simulink model "EHB_MOTOR"  (R2023b)
settings: Solver=FixedStepDiscrete  StartTime=0.0  StopTime=inf  FixedStep=0.0001  RelTol=1e-3  EnableMultiTasking=on
undefined symbols (not defined in the file): CAN_EHB_VCU0x125, CAN_EHB_VCU0x126, CAN_id0x120_Data, Cos_Table, Cos_Table1, EHB_DTC_status, R, Sin_BreakPoint, Sin_BreakPoint1, Sin_Table, Sin_Table1, T
libraries: simulink x30
(part 3 of 9)

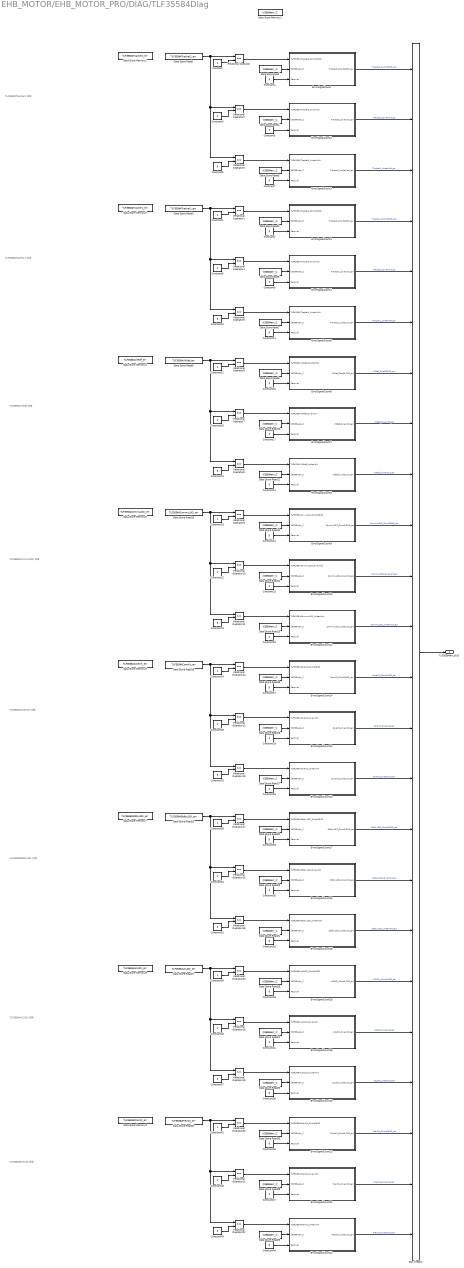
== system EHB_MOTOR/EHB_MOTOR_PRO/DIAG/TLF35584Diag ==
  note: TLF35584Tracker2故障
  note: TLF35584Tracker1故障
  note: TLF35584VltRef故障
  note: TLF35584CommuLDO故障
  note: TLF35584CoreVolt故障
  note: TLF35584StdbyLDO故障
  note: TLF35584uCLDO故障
  note: TLF35584PreVolt故障
  Bus Creator : BusCreator  Inputs=24
  Constant{,1,12,18,24,30,36,42} (8 alike) : Constant
  Constant{6,10,13,19,25,31,37,43} (8 alike) : Constant  Value=3
  Constant{2,4..5,7,9,11,14..15,17,20..21,23,26..27,29,32..33,35,38..39,41,44..45,47} (24 alike) : Constant  Value=0  OutDataTypeStr=uint8
  Constant{3,8,16,22,28,34,40,46} (8 alike) : Constant  Value=2
  Data Store Memory1 : DataStoreMemory  DataStoreName=ti35584err_C  ReadBeforeWriteMsg=warning  WriteAfterWriteMsg=warning  WriteAfterReadMsg=warning  ShowAdditionalParam=off  OutDataTypeStr=uint16
  Data Store Memory2 : DataStoreMemory  DataStoreName=TLF35584Tracker2_err  ReadBeforeWriteMsg=warning  WriteAfterWriteMsg=warning  WriteAfterReadMsg=warning  ShowAdditionalParam=off  OutDataTypeStr=uint8
  Data Store Memory3 : DataStoreMemory  DataStoreName=TLF35584Tracker1_err  ReadBeforeWriteMsg=warning  WriteAfterWriteMsg=warning  WriteAfterReadMsg=warning  ShowAdditionalParam=off  OutDataTypeStr=uint8
  Data Store Memory4 : DataStoreMemory  DataStoreName=TLF35584VltRef_err  ReadBeforeWriteMsg=warning  WriteAfterWriteMsg=warning  WriteAfterReadMsg=warning  ShowAdditionalParam=off  OutDataTypeStr=uint8
  Data Store Memory5 : DataStoreMemory  DataStoreName=TLF35584CommuLDO_err  ReadBeforeWriteMsg=warning  WriteAfterWriteMsg=warning  WriteAfterReadMsg=warning  ShowAdditionalParam=off  OutDataTypeStr=uint8
  Data Store Memory6 : DataStoreMemory  DataStoreName=TLF35584CoreVlt_err  ReadBeforeWriteMsg=warning  WriteAfterWriteMsg=warning  WriteAfterReadMsg=warning  ShowAdditionalParam=off  OutDataTypeStr=uint8
  Data Store Memory7 : DataStoreMemory  DataStoreName=TLF35584StdbyLDO_err  ReadBeforeWriteMsg=warning  WriteAfterWriteMsg=warning  WriteAfterReadMsg=warning  ShowAdditionalParam=off  OutDataTypeStr=uint8
  Data Store Memory8 : DataStoreMemory  DataStoreName=TLF35584uCLDO_err  ReadBeforeWriteMsg=warning  WriteAfterWriteMsg=warning  WriteAfterReadMsg=warning  ShowAdditionalParam=off  OutDataTypeStr=uint8
  Data Store Memory9 : DataStoreMemory  DataStoreName=TLF35584PreVolt_err  ReadBeforeWriteMsg=warning  WriteAfterWriteMsg=warning  WriteAfterReadMsg=warning  ShowAdditionalParam=off  OutDataTypeStr=uint8
  Data Store Read{,2,4..8,10..14,16..18,20..22,24..26,28..30} (24 alike) : DataStoreRead  DataStoreName=ti35584err_C  DataStoreElements=ti35584err_C  IndexOptions=Index vector (dialog)  Indices=1  OutputSizes=1
  Data Store Read1 : DataStoreRead  DataStoreName=TLF35584Tracker2_err  DataStoreElements=TLF35584Tracker2_err  IndexOptions=Index vector (dialog)  Indices=1  OutputSizes=1
  Data Store Read15 : DataStoreRead  DataStoreName=TLF35584CommuLDO_err  DataStoreElements=TLF35584CommuLDO_err  IndexOptions=Index vector (dialog)  Indices=1  OutputSizes=1
  Data Store Read19 : DataStoreRead  DataStoreName=TLF35584CoreVlt_err  DataStoreElements=TLF35584CoreVlt_err  IndexOptions=Index vector (dialog)  Indices=1  OutputSizes=1
  Data Store Read23 : DataStoreRead  DataStoreName=TLF35584StdbyLDO_err  DataStoreElements=TLF35584StdbyLDO_err  IndexOptions=Index vector (dialog)  Indices=1  OutputSizes=1
  Data Store Read27 : DataStoreRead  DataStoreName=TLF35584uCLDO_err  DataStoreElements=TLF35584uCLDO_err  IndexOptions=Index vector (dialog)  Indices=1  OutputSizes=1
  Data Store Read3 : DataStoreRead  DataStoreName=TLF35584Tracker1_err  DataStoreElements=TLF35584Tracker1_err  IndexOptions=Index vector (dialog)  Indices=1  OutputSizes=1
  Data Store Read31 : DataStoreRead  DataStoreName=TLF35584PreVolt_err  DataStoreElements=TLF35584PreVolt_err  IndexOptions=Index vector (dialog)  Indices=1  OutputSizes=1
  Data Store Read9 : DataStoreRead  DataStoreName=TLF35584VltRef_err  DataStoreElements=TLF35584VltRef_err  IndexOptions=Index vector (dialog)  Indices=1  OutputSizes=1
  ErrorSignalCount : Stateflow chart  TreatAsAtomicUnit=on
  ErrorSignalCount1 : Stateflow chart  TreatAsAtomicUnit=on
  ErrorSignalCount10 : Stateflow chart  TreatAsAtomicUnit=on
  ErrorSignalCount11 : Stateflow chart  TreatAsAtomicUnit=on
  ErrorSignalCount12 : Stateflow chart  TreatAsAtomicUnit=on
  ErrorSignalCount13 : Stateflow chart  TreatAsAtomicUnit=on
  ErrorSignalCount14 : Stateflow chart  TreatAsAtomicUnit=on
  ErrorSignalCount15 : Stateflow chart  TreatAsAtomicUnit=on
  ErrorSignalCount16 : Stateflow chart  TreatAsAtomicUnit=on
  ErrorSignalCount17 : Stateflow chart  TreatAsAtomicUnit=on
  ErrorSignalCount18 : Stateflow chart  TreatAsAtomicUnit=on
  ErrorSignalCount19 : Stateflow chart  TreatAsAtomicUnit=on
  ErrorSignalCount2 : Stateflow chart  TreatAsAtomicUnit=on
  ErrorSignalCount20 : Stateflow chart  TreatAsAtomicUnit=on
  ErrorSignalCount21 : Stateflow chart  TreatAsAtomicUnit=on
  ErrorSignalCount22 : Stateflow chart  TreatAsAtomicUnit=on
  ErrorSignalCount23 : Stateflow chart  TreatAsAtomicUnit=on
  ErrorSignalCount3 : Stateflow chart  TreatAsAtomicUnit=on
  ErrorSignalCount4 : Stateflow chart  TreatAsAtomicUnit=on
  ErrorSignalCount5 : Stateflow chart  TreatAsAtomicUnit=on
  ErrorSignalCount6 : Stateflow chart  TreatAsAtomicUnit=on
  ErrorSignalCount7 : Stateflow chart  TreatAsAtomicUnit=on
  ErrorSignalCount8 : Stateflow chart  TreatAsAtomicUnit=on
  ErrorSignalCount9 : Stateflow chart  TreatAsAtomicUnit=on
  Relational Operator{,1..23} (24 alike) : RelationalOperator  Operator===  OutDataTypeStr=boolean  RndMeth=Simplest  InputSameDT=off
  TLF35584err_BUS : Outport  VectorParamsAs1DForOutWhenUnconnected=off
  wires:
  Data Store Read/1 -> ErrorSignalCount/2(ti35584err_C)
  Constant4/1 -> ErrorSignalCount/3(Recover)
  Data Store Read1/1 -> Relational Operator/1, Relational Operator2/1, Relational Operator3/1
  Constant/1 -> Relational Operator/2
  Relational Operator/1 -> ErrorSignalCount/1(TLF35584Tracker2_Short2GND)
  Relational Operator1/1 -> ErrorSignalCount1/1(TLF35584Tracker1_Short2GND)
  Constant1/1 -> Relational Operator1/2
  Constant2/1 -> ErrorSignalCount1/3(Recover)
  Data Store Read2/1 -> ErrorSignalCount1/2(ti35584err_C)
  Constant3/1 -> Relational Operator2/2
  Constant5/1 -> ErrorSignalCount2/3(Recover)
  Data Store Read4/1 -> ErrorSignalCount2/2(ti35584err_C)
  Relational Operator2/1 -> ErrorSignalCount2/1(TLF35584Tracker2_OverVolt)
  Constant6/1 -> Relational Operator3/2
  Relational Operator3/1 -> ErrorSignalCount3/1(TLF35584Tracker2_UnderVolt)
  Data Store Read5/1 -> ErrorSignalCount3/2(ti35584err_C)
  Constant7/1 -> ErrorSignalCount3/3(Recover)
  Constant11/1 -> ErrorSignalCount5/3(Recover)
  Data Store Read7/1 -> ErrorSignalCount5/2(ti35584err_C)
  Relational Operator5/1 -> ErrorSignalCount5/1(TLF35584Tracker1_UnderVolt)
  Constant10/1 -> Relational Operator5/2
  Relational Operator4/1 -> ErrorSignalCount4/1(TLF35584Tracker1_OverVolt)
  Data Store Read6/1 -> ErrorSignalCount4/2(ti35584err_C)
  Constant9/1 -> ErrorSignalCount4/3(Recover)
  Constant8/1 -> Relational Operator4/2
  Data Store Read3/1 -> Relational Operator5/1, Relational Operator4/1, Relational Operator1/1
  Data Store Read9/1 -> Relational Operator6/1, Relational Operator7/1, Relational Operator8/1
  Constant16/1 -> Relational Operator7/2
  Constant17/1 -> ErrorSignalCount7/3(Recover)
  Data Store Read10/1 -> ErrorSignalCount7/2(ti35584err_C)
  Relational Operator7/1 -> ErrorSignalCount7/1(TLF35584VltRef_OverVolt)
  Constant13/1 -> Relational Operator8/2
  Relational Operator8/1 -> ErrorSignalCount8/1(TLF35584VltRef_UnderVolt)
  Data Store Read11/1 -> ErrorSignalCount8/2(ti35584err_C)
  Constant14/1 -> ErrorSignalCount8/3(Recover)
  Data Store Read8/1 -> ErrorSignalCount6/2(ti35584err_C)
  Constant15/1 -> ErrorSignalCount6/3(Recover)
  Constant12/1 -> Relational Operator6/2
  Relational Operator6/1 -> ErrorSignalCount6/1(TLF35584VltRef_Short2GND)
  Relational Operator9/1 -> ErrorSignalCount9/1(TLF35584CommuLDO_Short2GND)
  Constant18/1 -> Relational Operator9/2
  Constant21/1 -> ErrorSignalCount9/3(Recover)
  Data Store Read14/1 -> ErrorSignalCount9/2(ti35584err_C)
  Constant20/1 -> ErrorSignalCount11/3(Recover)
  Data Store Read13/1 -> ErrorSignalCount11/2(ti35584err_C)
  Relational Operator11/1 -> ErrorSignalCount11/1(TLF35584CommuLDO_UnderVolt)
  Constant19/1 -> Relational Operator11/2
  Relational Operator10/1 -> ErrorSignalCount10/1(TLF35584CommuLDO_OverVolt)
  Data Store Read12/1 -> ErrorSignalCount10/2(ti35584err_C)
  Constant23/1 -> ErrorSignalCount10/3(Recover)
  Constant22/1 -> Relational Operator10/2
  Data Store Read15/1 -> Relational Operator11/1, Relational Operator10/1, Relational Operator9/1
  Data Store Read19/1 -> Relational Operator14/1, Relational Operator13/1, Relational Operator12/1
  Constant28/1 -> Relational Operator12/2
  Constant29/1 -> ErrorSignalCount12/3(Recover)
  Data Store Read16/1 -> ErrorSignalCount12/2(ti35584err_C)
  Relational Operator12/1 -> ErrorSignalCount12/1(TLF35584CoreVlt_OverVolt)
  Constant25/1 -> Relational Operator13/2
  Relational Operator13/1 -> ErrorSignalCount13/1(TLF35584CoreVlt_UnderVolt)
  Data Store Read17/1 -> ErrorSignalCount13/2(ti35584err_C)
  Constant26/1 -> ErrorSignalCount13/3(Recover)
  Data Store Read18/1 -> ErrorSignalCount14/2(ti35584err_C)
  Constant27/1 -> ErrorSignalCount14/3(Recover)
  Constant24/1 -> Relational Operator14/2
  Relational Operator14/1 -> ErrorSignalCount14/1(TLF35584CoreVlt_Short2GND)
  Relational Operator17/1 -> ErrorSignalCount17/1(TLF35584StdbyLDO_Short2GND)
  Constant30/1 -> Relational Operator17/2
  Constant33/1 -> ErrorSignalCount17/3(Recover)
  Data Store Read22/1 -> ErrorSignalCount17/2(ti35584err_C)
  Constant32/1 -> ErrorSignalCount16/3(Recover)
  Data Store Read21/1 -> ErrorSignalCount16/2(ti35584err_C)
  Relational Operator16/1 -> ErrorSignalCount16/1(TLF35584StdbyLDO_UnderVolt)
  Constant31/1 -> Relational Operator16/2
  Relational Operator15/1 -> ErrorSignalCount15/1(TLF35584StdbyLDO_OverVolt)
  Data Store Read20/1 -> ErrorSignalCount15/2(ti35584err_C)
  Constant35/1 -> ErrorSignalCount15/3(Recover)
  Constant34/1 -> Relational Operator15/2
  Data Store Read23/1 -> Relational Operator16/1, Relational Operator15/1, Relational Operator17/1
  Data Store Read27/1 -> Relational Operator20/1, Relational Operator19/1, Relational Operator18/1
  Constant40/1 -> Relational Operator18/2
  Constant41/1 -> ErrorSignalCount18/3(Recover)
  Data Store Read24/1 -> ErrorSignalCount18/2(ti35584err_C)
  Relational Operator18/1 -> ErrorSignalCount18/1(TLF35584uCLDO_OverVolt)
  Constant37/1 -> Relational Operator19/2
  Relational Operator19/1 -> ErrorSignalCount19/1(TLF35584uCLDO_UnderVolt)
  Data Store Read25/1 -> ErrorSignalCount19/2(ti35584err_C)
  Constant38/1 -> ErrorSignalCount19/3(Recover)
  Data Store Read26/1 -> ErrorSignalCount20/2(ti35584err_C)
  Constant39/1 -> ErrorSignalCount20/3(Recover)
  Constant36/1 -> Relational Operator20/2
  Relational Operator20/1 -> ErrorSignalCount20/1(TLF35584uCLDO_Short2GND)
  Relational Operator23/1 -> ErrorSignalCount23/1(TLF35584PreVolt_Short2GND)
  Constant42/1 -> Relational Operator23/2
  Constant45/1 -> ErrorSignalCount23/3(Recover)
  Data Store Read30/1 -> ErrorSignalCount23/2(ti35584err_C)
  Constant44/1 -> ErrorSignalCount22/3(Recover)
  Data Store Read29/1 -> ErrorSignalCount22/2(ti35584err_C)
  Relational Operator22/1 -> ErrorSignalCount22/1(TLF35584PreVolt_UnderVolt)
  Constant43/1 -> Relational Operator22/2
  Relational Operator21/1 -> ErrorSignalCount21/1(TLF35584PreVolt_OverVolt)
  Data Store Read28/1 -> ErrorSignalCount21/2(ti35584err_C)
  Constant47/1 -> ErrorSignalCount21/3(Recover)
  Constant46/1 -> Relational Operator21/2
  Data Store Read31/1 -> Relational Operator22/1, Relational Operator21/1, Relational Operator23/1
  ErrorSignalCount/1(Tracker2_Short2GND_err) -> Bus Creator/1  "Tracker2_Short2GND_err"
  ErrorSignalCount2/1(Tracker2_OverVolt_err) -> Bus Creator/2  "Tracker2_OverVolt_err"
  ErrorSignalCount3/1(Tracker2_UnderVolt_err) -> Bus Creator/3  "Tracker2_UnderVolt_err"
  ErrorSignalCount1/1(Tracker1_Short2GND_err) -> Bus Creator/4  "Tracker1_Short2GND_err"
  ErrorSignalCount4/1(Tracker1_OverVolt_err) -> Bus Creator/5  "Tracker1_OverVolt_err"
  ErrorSignalCount5/1(Tracker1_UnderVolt_err) -> Bus Creator/6  "Tracker1_UnderVolt_err"
  ErrorSignalCount6/1(VltRef_Short2GND_err) -> Bus Creator/7  "VltRef_Short2GND_err"
  ErrorSignalCount7/1(VltRef_OverVolt_err) -> Bus Creator/8  "VltRef_OverVolt_err"
  ErrorSignalCount8/1(VltRef_UnderVolt_err) -> Bus Creator/9  "VltRef_UnderVolt_err"
  ErrorSignalCount9/1(CommuLDO_Short2GND_err) -> Bus Creator/10  "CommuLDO_Short2GND_err"
  ErrorSignalCount10/1(CommuLDO_OverVolt_err) -> Bus Creator/11  "CommuLDO_OverVolt_err"
  ErrorSignalCount11/1(CommuLDO_UnderVolt_err) -> Bus Creator/12  "CommuLDO_UnderVolt_err"
  ErrorSignalCount14/1(CoreVlt_Short2GND_err) -> Bus Creator/13  "CoreVlt_Short2GND_err"
  ErrorSignalCount12/1(CoreVlt_OverVolt_err) -> Bus Creator/14  "CoreVlt_OverVolt_err"
  ErrorSignalCount13/1(CoreVlt_UnderVolt_err) -> Bus Creator/15  "CoreVlt_UnderVolt_err"
  ErrorSignalCount17/1(StdbyLDO_Short2GND_err) -> Bus Creator/16  "StdbyLDO_Short2GND_err"
  ErrorSignalCount15/1(StdbyLDO_OverVolt_err) -> Bus Creator/17  "StdbyLDO_OverVolt_err"
  ErrorSignalCount16/1(StdbyLDO_UnderVolt_err) -> Bus Creator/18  "StdbyLDO_UnderVolt_err"
  ErrorSignalCount20/1(uCLDO_Short2GND_err) -> Bus Creator/19  "uCLDO_Short2GND_err"
  ErrorSignalCount18/1(uCLDO_OverVolt_err) -> Bus Creator/20  "uCLDO_OverVolt_err"
  ErrorSignalCount19/1(uCLDO_UnderVolt_err) -> Bus Creator/21  "uCLDO_UnderVolt_err"
  ErrorSignalCount23/1(PreVolt_Short2GND_err) -> Bus Creator/22  "PreVolt_Short2GND_err"
  ErrorSignalCount21/1(PreVolt_OverVolt_err) -> Bus Creator/23  "PreVolt_OverVolt_err"
  ErrorSignalCount22/1(PreVolt_UnderVolt_err) -> Bus Creator/24  "PreVolt_UnderVolt_err"
  Bus Creator/1 -> TLF35584err_BUS/1

== system EHB_MOTOR/EHB_MOTOR_PRO/DIAG/TempDiag ==
  note: 200ms
  note: 温度传感器故障
  TempSensor : Inport
  Chart : Stateflow chart  TreatAsAtomicUnit=on
  Subsystem1 : Subsystem
  TempSensorOverride : Outport  VectorParamsAs1DForOutWhenUnconnected=off
  wires:
  Subsystem1/1(Out1) -> TempSensorOverride/1
  TempSensor/1 -> Subsystem1/1(In1)
  Chart/1(task_200ms()) -> Subsystem1/Trigger

== system EHB_MOTOR/EHB_MOTOR_PRO/DIAG/UDS_interface ==
  DiagBUS : Inport
  Bus Selector : BusSelector  OutputSignals=EHBVoltageLow2
  Bus Selector1 : BusSelector  OutputSignals=EHBVoltageHigh2
  Bus Selector10 : BusSelector  OutputSignals=5vErr
  Bus Selector12 : BusSelector  OutputSignals=Chip7189_err
  Bus Selector14 : BusSelector  OutputSignals=PressureFlowERR2
  Bus Selector2 : BusSelector  OutputSignals=TempSensorOverride
  Bus Selector3 : BusSelector  OutputSignals=PressureSensorERR
  Bus Selector4 : BusSelector  OutputSignals=CurrentSensorUOverride,CurrentSensorVOverride,CurrentSensorWOverride
  Bus Selector5 : BusSelector  OutputSignals=TLF35584err_BUS.Tracker2_Short2GND_err,TLF35584err_BUS.Tracker2_OverVolt_err,TLF35584err_BUS.Tracker2_UnderVolt_err,TLF35584err_BUS.Tracker1_Short2GND_err,TLF35584err_BUS.Tracker1_OverVolt_err,TLF35584err_BUS.Tracker1_UnderVolt_err,TLF35584err_BUS.VltRef_Short2GND_err,TLF35584err_BUS.VltRef_OverVolt_err,TLF35584err_BUS.VltRef_UnderVolt_err,TLF35584err_BUS.CommuLDO_Short2GND_err,TLF35584err_BUS.CommuLDO_OverVolt_err,TLF35584err_BUS.CommuLDO_UnderVolt_err,TLF35584err_BUS.CoreVlt_Short2GND_err,TLF35584err_BUS.CoreVlt_OverVolt_err,TLF35584err_BUS.CoreVlt_UnderVolt_err,TLF35584err_BUS.StdbyLDO_Short2GND_err,TLF35584err_BUS.StdbyLDO_OverVolt_err,TLF35584err_BUS.StdbyLDO_UnderVolt_err,TLF35584err_BUS.uCLDO_Short2GND_err,TLF35584err_BUS.uCLDO_OverVolt_err,TLF35584err_BUS.uCLDO_UnderVolt_err,TLF35584err_BUS.PreVolt_Short2GND_err,TLF35584err_BUS.PreVolt_OverVolt_err,TLF35584err_BUS.PreVolt_UnderVolt_err
  Bus Selector6 : BusSelector  OutputSignals=AngleSensorSignalOverride
  Bus Selector7 : BusSelector  OutputSignals=AngleSensorSignalLost
  Bus Selector8 : BusSelector  OutputSignals=Mot_locked_err
  Constant{,1..10,12..15} (15 alike) : Constant  Value=0
  DTC_pack : Stateflow chart  TreatAsAtomicUnit=on
  Data Store Memory2 : DataStoreMemory  DataStoreName=Clear_DTC  ReadBeforeWriteMsg=warning  WriteAfterWriteMsg=warning  WriteAfterReadMsg=warning  ShowAdditionalParam=off  OutDataTypeStr=uint8
  Data Store Read2 : DataStoreRead  DataStoreName=Clear_DTC  DataStoreElements=Clear_DTC  IndexOptions=Index vector (dialog)  Indices=1  OutputSizes=1
  Logical Operator : Logic  Operator=OR  Inputs=3  AllPortsSameDT=off  OutDataTypeStr=boolean
  EHB_DTC : Outport  VectorParamsAs1DForOutWhenUnconnected=off
  wires:
  DiagBUS/1 -> Bus Selector/1, Bus Selector1/1, Bus Selector2/1, Bus Selector3/1, Bus Selector6/1, Bus Selector7/1, Bus Selector8/1, Bus Selector10/1, Bus Selector12/1, Bus Selector14/1, Bus Selector5/1, Bus Selector4/1
  DTC_pack/1(EHB_DTC) -> EHB_DTC/1
  Bus Selector/1 -> DTC_pack/1(minBAT)  "<EHBVoltageLow2>"
  Bus Selector1/1 -> DTC_pack/2(maxBAT)  "<EHBVoltageHigh2>"
  Bus Selector2/1 -> DTC_pack/3(overTemp)  "<TempSensorOverride>"
  Bus Selector6/1 -> DTC_pack/7(errAngleSensor)  "<AngleSensorSignalOverride>"
  Bus Selector7/1 -> DTC_pack/8(noAngleSensor)  "<AngleSensorSignalLost>"
  Constant/1 -> DTC_pack/9(unCalAngleSensor)
  Constant2/1 -> DTC_pack/11(noPreSensor)
  Constant1/1 -> DTC_pack/10(errPreSensor)
  Constant3/1 -> DTC_pack/12(unCalPreSensor)
  Constant4/1 -> DTC_pack/13(errTqSensor)
  Constant5/1 -> DTC_pack/14(noTqSensor)
  Constant6/1 -> DTC_pack/15(unCalTqSensor)
  Bus Selector8/1 -> DTC_pack/16(errMotorloop)  "<Mot_locked_err>"
  Bus Selector10/1 -> DTC_pack/18(err5vOUT)  "<5vErr>"
  Bus Selector12/1 -> DTC_pack/21(errA3941)  "<Chip7189_err>"
  Bus Selector14/1 -> DTC_pack/23(errResponce)  "<PressureFlowERR2>"
  Constant7/1 -> DTC_pack/24(errCANHW)
  Constant8/1 -> DTC_pack/25(CANDataLoss)
  Constant9/1 -> DTC_pack/26(BUSOFF)
  Data Store Read2/1 -> DTC_pack/27(Clear_minBAT_req)
  Constant10/1 -> DTC_pack/4(errTempSensor)
  Logical Operator/1 -> DTC_pack/5(overCurrent)
  Bus Selector4/1 -> Logical Operator/1  "<CurrentSensorUOverride>"
  Bus Selector4/2 -> Logical Operator/2  "<CurrentSensorVOverride>"
  Bus Selector4/3 -> Logical Operator/3  "<CurrentSensorWOverride>"
  Constant12/1 -> DTC_pack/17(errPreCtl)
  Constant13/1 -> DTC_pack/19(errHSO1)
  Constant14/1 -> DTC_pack/20(errHSO2)
  Constant15/1 -> DTC_pack/22(errPWM)
  Bus Selector3/1 -> DTC_pack/6(errCurSensor)  "<PressureSensorERR>"
  Bus Selector5/1 -> DTC_pack/28(Tracker2_Short2GND_err)  "<Tracker2_Short2GND_err>"
  Bus Selector5/2 -> DTC_pack/29(Tracker2_OverVolt_err)  "<Tracker2_OverVolt_err>"
  Bus Selector5/3 -> DTC_pack/30(Tracker2_UnderVolt_err)  "<Tracker2_UnderVolt_err>"
  Bus Selector5/4 -> DTC_pack/31(Tracker1_Short2GND_err)  "<Tracker1_Short2GND_err>"
  Bus Selector5/5 -> DTC_pack/32(Tracker1_OverVolt_err)  "<Tracker1_OverVolt_err>"
  Bus Selector5/6 -> DTC_pack/33(Tracker1_UnderVolt_err)  "<Tracker1_UnderVolt_err>"
  Bus Selector5/7 -> DTC_pack/34(VltRef_Short2GND_err)  "<VltRef_Short2GND_err>"
  Bus Selector5/8 -> DTC_pack/35(VltRef_OverVolt_err)  "<VltRef_OverVolt_err>"
  Bus Selector5/9 -> DTC_pack/36(VltRef_UnderVolt_err)  "<VltRef_UnderVolt_err>"
  Bus Selector5/10 -> DTC_pack/37(CommuLDO_Short2GND_err)  "<CommuLDO_Short2GND_err>"
  Bus Selector5/11 -> DTC_pack/38(CommuLDO_OverVolt_err)  "<CommuLDO_OverVolt_err>"
  Bus Selector5/12 -> DTC_pack/39(CommuLDO_UnderVolt_err)  "<CommuLDO_UnderVolt_err>"
  Bus Selector5/13 -> DTC_pack/40(CoreVlt_Short2GND_err)  "<CoreVlt_Short2GND_err>"
  Bus Selector5/14 -> DTC_pack/41(CoreVlt_OverVolt_err)  "<CoreVlt_OverVolt_err>"
  Bus Selector5/15 -> DTC_pack/42(CoreVlt_UnderVolt_err)  "<CoreVlt_UnderVolt_err>"
  Bus Selector5/16 -> DTC_pack/43(StdbyLDO_Short2GND_err)  "<StdbyLDO_Short2GND_err>"
  Bus Selector5/17 -> DTC_pack/44(StdbyLDO_OverVolt_err)  "<StdbyLDO_OverVolt_err>"
  Bus Selector5/18 -> DTC_pack/45(StdbyLDO_UnderVolt_err)  "<StdbyLDO_UnderVolt_err>"
  Bus Selector5/19 -> DTC_pack/46(uCLDO_Short2GND_err)  "<uCLDO_Short2GND_err>"
  Bus Selector5/20 -> DTC_pack/47(uCLDO_OverVolt_err)  "<uCLDO_OverVolt_err>"
  Bus Selector5/21 -> DTC_pack/48(uCLDO_UnderVolt_err)  "<uCLDO_UnderVolt_err>"
  Bus Selector5/22 -> DTC_pack/49(PreVolt_Short2GND_err)  "<PreVolt_Short2GND_err>"
  Bus Selector5/23 -> DTC_pack/50(PreVolt_OverVolt_err)  "<PreVolt_OverVolt_err>"
  Bus Selector5/24 -> DTC_pack/51(PreVolt_UnderVolt_err)  "<PreVolt_UnderVolt_err>"

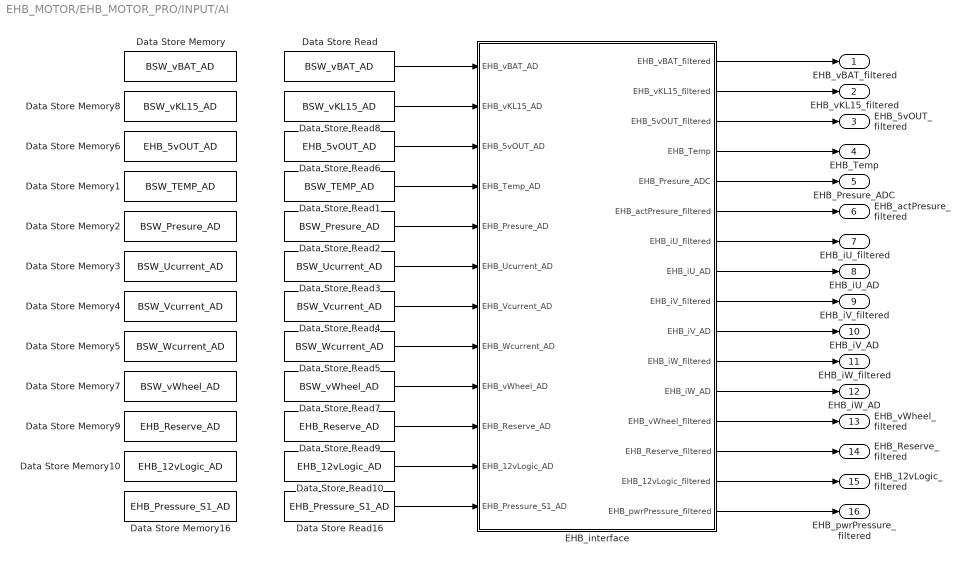
== system EHB_MOTOR/EHB_MOTOR_PRO/INPUT/AI ==
  Data Store Memory : DataStoreMemory  DataStoreName=BSW_vBAT_AD  ReadBeforeWriteMsg=warning  WriteAfterWriteMsg=warning  WriteAfterReadMsg=warning  ShowAdditionalParam=off  OutDataTypeStr=uint16
  Data Store Memory1 : DataStoreMemory  DataStoreName=BSW_TEMP_AD  ReadBeforeWriteMsg=warning  WriteAfterWriteMsg=warning  WriteAfterReadMsg=warning  ShowAdditionalParam=off  OutDataTypeStr=uint16
  Data Store Memory10 : DataStoreMemory  DataStoreName=EHB_12vLogic_AD  ReadBeforeWriteMsg=warning  WriteAfterWriteMsg=warning  WriteAfterReadMsg=warning  ShowAdditionalParam=off  OutDataTypeStr=uint16
  Data Store Memory16 : DataStoreMemory  DataStoreName=EHB_Pressure_S1_AD  ReadBeforeWriteMsg=warning  WriteAfterWriteMsg=warning  WriteAfterReadMsg=warning  ShowAdditionalParam=off  OutDataTypeStr=uint16
  Data Store Memory2 : DataStoreMemory  DataStoreName=BSW_Presure_AD  ReadBeforeWriteMsg=warning  WriteAfterWriteMsg=warning  WriteAfterReadMsg=warning  ShowAdditionalParam=off  OutDataTypeStr=uint16
  Data Store Memory3 : DataStoreMemory  DataStoreName=BSW_Ucurrent_AD  ReadBeforeWriteMsg=warning  WriteAfterWriteMsg=warning  WriteAfterReadMsg=warning  ShowAdditionalParam=off  OutDataTypeStr=uint16
  Data Store Memory4 : DataStoreMemory  DataStoreName=BSW_Vcurrent_AD  ReadBeforeWriteMsg=warning  WriteAfterWriteMsg=warning  WriteAfterReadMsg=warning  ShowAdditionalParam=off  OutDataTypeStr=uint16
  Data Store Memory5 : DataStoreMemory  DataStoreName=BSW_Wcurrent_AD  ReadBeforeWriteMsg=warning  WriteAfterWriteMsg=warning  WriteAfterReadMsg=warning  ShowAdditionalParam=off  OutDataTypeStr=uint16
  Data Store Memory6 : DataStoreMemory  DataStoreName=EHB_5vOUT_AD  ReadBeforeWriteMsg=warning  WriteAfterWriteMsg=warning  WriteAfterReadMsg=warning  ShowAdditionalParam=off  OutDataTypeStr=uint16
  Data Store Memory7 : DataStoreMemory  DataStoreName=BSW_vWheel_AD  ReadBeforeWriteMsg=warning  WriteAfterWriteMsg=warning  WriteAfterReadMsg=warning  ShowAdditionalParam=off  OutDataTypeStr=uint16
  Data Store Memory8 : DataStoreMemory  DataStoreName=BSW_vKL15_AD  ReadBeforeWriteMsg=warning  WriteAfterWriteMsg=warning  WriteAfterReadMsg=warning  ShowAdditionalParam=off  OutDataTypeStr=uint16
  Data Store Memory9 : DataStoreMemory  DataStoreName=EHB_Reserve_AD  ReadBeforeWriteMsg=warning  WriteAfterWriteMsg=warning  WriteAfterReadMsg=warning  ShowAdditionalParam=off  OutDataTypeStr=uint16
  Data Store Read : DataStoreRead  DataStoreName=BSW_vBAT_AD  DataStoreElements=BSW_vBAT_AD  IndexOptions=Index vector (dialog)  Indices=1  OutputSizes=1
  Data Store Read1 : DataStoreRead  DataStoreName=BSW_TEMP_AD  DataStoreElements=BSW_TEMP_AD  IndexOptions=Index vector (dialog)  Indices=1  OutputSizes=1
  Data Store Read10 : DataStoreRead  DataStoreName=EHB_12vLogic_AD  DataStoreElements=EHB_12vLogic_AD  IndexOptions=Index vector (dialog)  Indices=1  OutputSizes=1
  Data Store Read16 : DataStoreRead  DataStoreName=EHB_Pressure_S1_AD  DataStoreElements=EHB_Pressure_S1_AD  IndexOptions=Index vector (dialog)  Indices=1  OutputSizes=1
  Data Store Read2 : DataStoreRead  DataStoreName=BSW_Presure_AD  DataStoreElements=BSW_Presure_AD  IndexOptions=Index vector (dialog)  Indices=1  OutputSizes=1
  Data Store Read3 : DataStoreRead  DataStoreName=BSW_Ucurrent_AD  DataStoreElements=BSW_Ucurrent_AD  IndexOptions=Index vector (dialog)  Indices=1  OutputSizes=1
  Data Store Read4 : DataStoreRead  DataStoreName=BSW_Vcurrent_AD  DataStoreElements=BSW_Vcurrent_AD  IndexOptions=Index vector (dialog)  Indices=1  OutputSizes=1
  Data Store Read5 : DataStoreRead  DataStoreName=BSW_Wcurrent_AD  DataStoreElements=BSW_Wcurrent_AD  IndexOptions=Index vector (dialog)  Indices=1  OutputSizes=1
  Data Store Read6 : DataStoreRead  DataStoreName=EHB_5vOUT_AD  DataStoreElements=EHB_5vOUT_AD  IndexOptions=Index vector (dialog)  Indices=1  OutputSizes=1
  Data Store Read7 : DataStoreRead  DataStoreName=BSW_vWheel_AD  DataStoreElements=BSW_vWheel_AD  IndexOptions=Index vector (dialog)  Indices=1  OutputSizes=1
  Data Store Read8 : DataStoreRead  DataStoreName=BSW_vKL15_AD  DataStoreElements=BSW_vKL15_AD  IndexOptions=Index vector (dialog)  Indices=1  OutputSizes=1
  Data Store Read9 : DataStoreRead  DataStoreName=EHB_Reserve_AD  DataStoreElements=EHB_Reserve_AD  IndexOptions=Index vector (dialog)  Indices=1  OutputSizes=1
  EHB_interface : Subsystem
  EHB_vBAT_filtered : Outport  VectorParamsAs1DForOutWhenUnconnected=off
  EHB_vKL15_filtered : Outport  Port=2  VectorParamsAs1DForOutWhenUnconnected=off
  EHB_5vOUT_filtered : Outport  Port=3  VectorParamsAs1DForOutWhenUnconnected=off
  EHB_Temp : Outport  Port=4  VectorParamsAs1DForOutWhenUnconnected=off
  EHB_Presure_ADC : Outport  Port=5  VectorParamsAs1DForOutWhenUnconnected=off
  EHB_actPresure_filtered : Outport  Port=6  VectorParamsAs1DForOutWhenUnconnected=off
  EHB_iU_filtered : Outport  Port=7  VectorParamsAs1DForOutWhenUnconnected=off
  EHB_iU_AD : Outport  Port=8  VectorParamsAs1DForOutWhenUnconnected=off
  EHB_iV_filtered : Outport  Port=9  VectorParamsAs1DForOutWhenUnconnected=off
  EHB_iV_AD : Outport  Port=10  VectorParamsAs1DForOutWhenUnconnected=off
  EHB_iW_filtered : Outport  Port=11  VectorParamsAs1DForOutWhenUnconnected=off
  EHB_iW_AD : Outport  Port=12  VectorParamsAs1DForOutWhenUnconnected=off
  EHB_vWheel_filtered : Outport  Port=13  VectorParamsAs1DForOutWhenUnconnected=off
  EHB_Reserve_filtered : Outport  Port=14  VectorParamsAs1DForOutWhenUnconnected=off
  EHB_12vLogic_filtered : Outport  Port=15  VectorParamsAs1DForOutWhenUnconnected=off
  EHB_pwrPressure_filtered : Outport  Port=16  VectorParamsAs1DForOutWhenUnconnected=off
  wires:
  Data Store Read8/1 -> EHB_interface/2(EHB_vKL15_AD)
  Data Store Read1/1 -> EHB_interface/4(EHB_Temp_AD)
  Data Store Read/1 -> EHB_interface/1(EHB_vBAT_AD)
  Data Store Read6/1 -> EHB_interface/3(EHB_5vOUT_AD)
  Data Store Read2/1 -> EHB_interface/5(EHB_Presure_AD)
  Data Store Read3/1 -> EHB_interface/6(EHB_Ucurrent_AD)
  Data Store Read4/1 -> EHB_interface/7(EHB_Vcurrent_AD)
  Data Store Read5/1 -> EHB_interface/8(EHB_Wcurrent_AD)
  Data Store Read7/1 -> EHB_interface/9(EHB_vWheel_AD)
  Data Store Read9/1 -> EHB_interface/10(EHB_Reserve_AD)
  Data Store Read10/1 -> EHB_interface/11(EHB_12vLogic_AD)
  Data Store Read16/1 -> EHB_interface/12(EHB_Pressure_S1_AD)
  EHB_interface/5(EHB_Presure_ADC) -> EHB_Presure_ADC/1
  EHB_interface/8(EHB_iU_AD) -> EHB_iU_AD/1
  EHB_interface/10(EHB_iV_AD) -> EHB_iV_AD/1
  EHB_interface/12(EHB_iW_AD) -> EHB_iW_AD/1
  EHB_interface/4(EHB_Temp) -> EHB_Temp/1
  EHB_interface/3(EHB_5vOUT_filtered) -> EHB_5vOUT_filtered/1
  EHB_interface/2(EHB_vKL15_filtered) -> EHB_vKL15_filtered/1
  EHB_interface/1(EHB_vBAT_filtered) -> EHB_vBAT_filtered/1
  EHB_interface/6(EHB_actPresure_filtered) -> EHB_actPresure_filtered/1
  EHB_interface/7(EHB_iU_filtered) -> EHB_iU_filtered/1
  EHB_interface/9(EHB_iV_filtered) -> EHB_iV_filtered/1
  EHB_interface/11(EHB_iW_filtered) -> EHB_iW_filtered/1
  EHB_interface/13(EHB_vWheel_filtered) -> EHB_vWheel_filtered/1
  EHB_interface/14(EHB_Reserve_filtered) -> EHB_Reserve_filtered/1
  EHB_interface/15(EHB_12vLogic_filtered) -> EHB_12vLogic_filtered/1
  EHB_interface/16(EHB_pwrPressure_filtered) -> EHB_pwrPressure_filtered/1

== system EHB_MOTOR/EHB_MOTOR_PRO/INPUT/CAN ==
  0x120 : Stateflow chart  TreatAsAtomicUnit=on
  Data Store Memory : DataStoreMemory  DataStoreName=EHB_reqPresure  ReadBeforeWriteMsg=warning  WriteAfterWriteMsg=warning  WriteAfterReadMsg=warning  ShowAdditionalParam=off  OutDataTypeStr=single
  Data Store Memory1 : DataStoreMemory  DataStoreName=VCU_BrakingEnable  ReadBeforeWriteMsg=warning  WriteAfterWriteMsg=warning  WriteAfterReadMsg=warning  ShowAdditionalParam=off  OutDataTypeStr=uint8
  Data Store Memory5 : DataStoreMemory  DataStoreName=CAN_id0x120_Data  ReadBeforeWriteMsg=warning  WriteAfterWriteMsg=warning  WriteAfterReadMsg=warning  ShowAdditionalParam=off  OutDataTypeStr=uint8  Dimensions=8
  Data Store Read5 : DataStoreRead  DataStoreName=CAN_id0x120_Data  DataStoreElements=CAN_id0x120_Data(:)  IndexOptions=Index vector (dialog)  Indices=1  OutputSizes=1
  Data Store Write : DataStoreWrite  DataStoreName=EHB_reqPresure  DataStoreElements=EHB_reqPresure  IndexOptions=Index vector (dialog)  Indices=1  OutputSizes=1
  Data Store Write1 : DataStoreWrite  DataStoreName=VCU_BrakingEnable  DataStoreElements=VCU_BrakingEnable  IndexOptions=Index vector (dialog)  Indices=1  OutputSizes=1
  VCU_BrakingEnable : Outport  VectorParamsAs1DForOutWhenUnconnected=off
  VCU_ParkingBrakeActive : Outport  Port=2  VectorParamsAs1DForOutWhenUnconnected=off
  VCU_Brake_AimPressure : Outport  Port=3  VectorParamsAs1DForOutWhenUnconnected=off
  VCU_RollingCounter : Outport  Port=4  VectorParamsAs1DForOutWhenUnconnected=off
  VCU_Checksum : Outport  Port=5  VectorParamsAs1DForOutWhenUnconnected=off
  wires:
  0x120/1(BrakingEnable) -> Data Store Write1/1, VCU_BrakingEnable/1
  0x120/2(ParkingBrakeActive) -> VCU_ParkingBrakeActive/1
  0x120/3(Brake_AimPressure) -> VCU_Brake_AimPressure/1, Data Store Write/1
  0x120/4(RollingCounter) -> VCU_RollingCounter/1
  0x120/5(Checksum) -> VCU_Checksum/1
  Data Store Read5/1 -> 0x120/1(CAN_id0x120_Data)

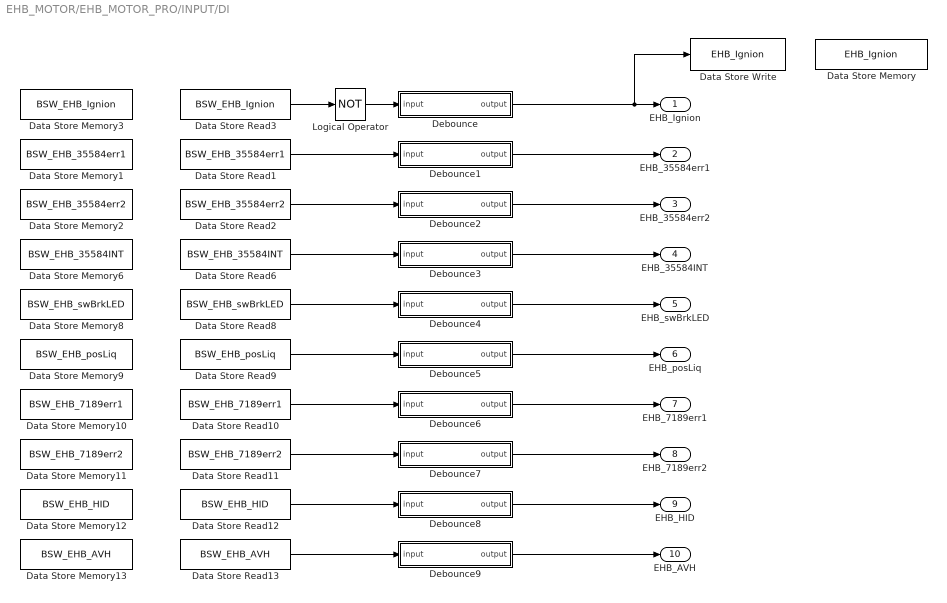
== system EHB_MOTOR/EHB_MOTOR_PRO/INPUT/DI ==
  Data Store Memory : DataStoreMemory  DataStoreName=EHB_Ignion  ReadBeforeWriteMsg=warning  WriteAfterWriteMsg=warning  WriteAfterReadMsg=warning  ShowAdditionalParam=off  OutDataTypeStr=boolean
  Data Store Memory1 : DataStoreMemory  DataStoreName=BSW_EHB_35584err1  ReadBeforeWriteMsg=warning  WriteAfterWriteMsg=warning  WriteAfterReadMsg=warning  ShowAdditionalParam=off  OutDataTypeStr=boolean
  Data Store Memory10 : DataStoreMemory  DataStoreName=BSW_EHB_7189err1  ReadBeforeWriteMsg=warning  WriteAfterWriteMsg=warning  WriteAfterReadMsg=warning  ShowAdditionalParam=off  OutDataTypeStr=boolean
  Data Store Memory11 : DataStoreMemory  DataStoreName=BSW_EHB_7189err2  ReadBeforeWriteMsg=warning  WriteAfterWriteMsg=warning  WriteAfterReadMsg=warning  ShowAdditionalParam=off  OutDataTypeStr=boolean
  Data Store Memory12 : DataStoreMemory  DataStoreName=BSW_EHB_HID  ReadBeforeWriteMsg=warning  WriteAfterWriteMsg=warning  WriteAfterReadMsg=warning  ShowAdditionalParam=off  OutDataTypeStr=boolean
  Data Store Memory13 : DataStoreMemory  DataStoreName=BSW_EHB_AVH  ReadBeforeWriteMsg=warning  WriteAfterWriteMsg=warning  WriteAfterReadMsg=warning  ShowAdditionalParam=off  OutDataTypeStr=boolean
  Data Store Memory2 : DataStoreMemory  DataStoreName=BSW_EHB_35584err2  ReadBeforeWriteMsg=warning  WriteAfterWriteMsg=warning  WriteAfterReadMsg=warning  ShowAdditionalParam=off  OutDataTypeStr=boolean
  Data Store Memory3 : DataStoreMemory  DataStoreName=BSW_EHB_Ignion  ReadBeforeWriteMsg=warning  WriteAfterWriteMsg=warning  WriteAfterReadMsg=warning  ShowAdditionalParam=off  OutDataTypeStr=boolean
  Data Store Memory6 : DataStoreMemory  DataStoreName=BSW_EHB_35584INT  ReadBeforeWriteMsg=warning  WriteAfterWriteMsg=warning  WriteAfterReadMsg=warning  ShowAdditionalParam=off  OutDataTypeStr=boolean
  Data Store Memory8 : DataStoreMemory  DataStoreName=BSW_EHB_swBrkLED  ReadBeforeWriteMsg=warning  WriteAfterWriteMsg=warning  WriteAfterReadMsg=warning  ShowAdditionalParam=off  OutDataTypeStr=boolean
  Data Store Memory9 : DataStoreMemory  DataStoreName=BSW_EHB_posLiq  ReadBeforeWriteMsg=warning  WriteAfterWriteMsg=warning  WriteAfterReadMsg=warning  ShowAdditionalParam=off  OutDataTypeStr=boolean
  Data Store Read1 : DataStoreRead  DataStoreName=BSW_EHB_35584err1  DataStoreElements=BSW_EHB_35584err1  IndexOptions=Index vector (dialog)  Indices=1  OutputSizes=1
  Data Store Read10 : DataStoreRead  DataStoreName=BSW_EHB_7189err1  DataStoreElements=BSW_EHB_7189err1  IndexOptions=Index vector (dialog)  Indices=1  OutputSizes=1
  Data Store Read11 : DataStoreRead  DataStoreName=BSW_EHB_7189err2  DataStoreElements=BSW_EHB_7189err2  IndexOptions=Index vector (dialog)  Indices=1  OutputSizes=1
  Data Store Read12 : DataStoreRead  DataStoreName=BSW_EHB_HID  DataStoreElements=BSW_EHB_HID  IndexOptions=Index vector (dialog)  Indices=1  OutputSizes=1
  Data Store Read13 : DataStoreRead  DataStoreName=BSW_EHB_AVH  DataStoreElements=BSW_EHB_AVH  IndexOptions=Index vector (dialog)  Indices=1  OutputSizes=1
  Data Store Read2 : DataStoreRead  DataStoreName=BSW_EHB_35584err2  DataStoreElements=BSW_EHB_35584err2  IndexOptions=Index vector (dialog)  Indices=1  OutputSizes=1
  Data Store Read3 : DataStoreRead  DataStoreName=BSW_EHB_Ignion  DataStoreElements=BSW_EHB_Ignion  IndexOptions=Index vector (dialog)  Indices=1  OutputSizes=1
  Data Store Read6 : DataStoreRead  DataStoreName=BSW_EHB_35584INT  DataStoreElements=BSW_EHB_35584INT  IndexOptions=Index vector (dialog)  Indices=1  OutputSizes=1
  Data Store Read8 : DataStoreRead  DataStoreName=BSW_EHB_swBrkLED  DataStoreElements=BSW_EHB_swBrkLED  IndexOptions=Index vector (dialog)  Indices=1  OutputSizes=1
  Data Store Read9 : DataStoreRead  DataStoreName=BSW_EHB_posLiq  DataStoreElements=BSW_EHB_posLiq  IndexOptions=Index vector (dialog)  Indices=1  OutputSizes=1
  Data Store Write : DataStoreWrite  DataStoreName=EHB_Ignion  DataStoreElements=EHB_Ignion  IndexOptions=Index vector (dialog)  Indices=1  OutputSizes=1
  Debounce : Stateflow chart  TreatAsAtomicUnit=on
  Debounce1 : Stateflow chart  TreatAsAtomicUnit=on
  Debounce2 : Stateflow chart  TreatAsAtomicUnit=on
  Debounce3 : Stateflow chart  TreatAsAtomicUnit=on
  Debounce4 : Stateflow chart  TreatAsAtomicUnit=on
  Debounce5 : Stateflow chart  TreatAsAtomicUnit=on
  Debounce6 : Stateflow chart  TreatAsAtomicUnit=on
  Debounce7 : Stateflow chart  TreatAsAtomicUnit=on
  Debounce8 : Stateflow chart  TreatAsAtomicUnit=on
  Debounce9 : Stateflow chart  TreatAsAtomicUnit=on
  Logical Operator : Logic  Operator=NOT  AllPortsSameDT=off  OutDataTypeStr=boolean
  EHB_Ignion : Outport  VectorParamsAs1DForOutWhenUnconnected=off
  EHB_35584err1 : Outport  Port=2  VectorParamsAs1DForOutWhenUnconnected=off
  EHB_35584err2 : Outport  Port=3  VectorParamsAs1DForOutWhenUnconnected=off
  EHB_35584INT : Outport  Port=4  VectorParamsAs1DForOutWhenUnconnected=off
  EHB_swBrkLED : Outport  Port=5  VectorParamsAs1DForOutWhenUnconnected=off
  EHB_posLiq : Outport  Port=6  VectorParamsAs1DForOutWhenUnconnected=off
  EHB_7189err1 : Outport  Port=7  VectorParamsAs1DForOutWhenUnconnected=off
  EHB_7189err2 : Outport  Port=8  VectorParamsAs1DForOutWhenUnconnected=off
  EHB_HID : Outport  Port=9  VectorParamsAs1DForOutWhenUnconnected=off
  EHB_AVH : Outport  Port=10  VectorParamsAs1DForOutWhenUnconnected=off
  wires:
  Data Store Read1/1 -> Debounce1/1(input)
  Data Store Read10/1 -> Debounce6/1(input)
  Data Store Read6/1 -> Debounce3/1(input)
  Data Store Read12/1 -> Debounce8/1(input)
  Data Store Read2/1 -> Debounce2/1(input)
  Data Store Read8/1 -> Debounce4/1(input)
  Data Store Read9/1 -> Debounce5/1(input)
  Data Store Read11/1 -> Debounce7/1(input)
  Data Store Read13/1 -> Debounce9/1(input)
  Debounce1/1(output) -> EHB_35584err1/1
  Debounce2/1(output) -> EHB_35584err2/1
  Debounce3/1(output) -> EHB_35584INT/1
  Debounce4/1(output) -> EHB_swBrkLED/1
  Debounce5/1(output) -> EHB_posLiq/1
  Debounce6/1(output) -> EHB_7189err1/1
  Debounce7/1(output) -> EHB_7189err2/1
  Debounce8/1(output) -> EHB_HID/1
  Debounce9/1(output) -> EHB_AVH/1
  Debounce/1(output) -> Data Store Write/1, EHB_Ignion/1
  Data Store Read3/1 -> Logical Operator/1
  Logical Operator/1 -> Debounce/1(input)

== system EHB_MOTOR/EHB_MOTOR_PRO/INPUT/MOTOR ==
  Data Store Memory4 : DataStoreMemory  DataStoreName=EHBMotor_Pos_AD  ReadBeforeWriteMsg=warning  WriteAfterWriteMsg=warning  WriteAfterReadMsg=warning  ShowAdditionalParam=off  OutDataTypeStr=uint16
  Data Store Memory7 : DataStoreMemory  DataStoreName=EHBMotor_PWM  ReadBeforeWriteMsg=warning  WriteAfterWriteMsg=warning  WriteAfterReadMsg=warning  ShowAdditionalParam=off  OutDataTypeStr=double
  Data Store Read4 : DataStoreRead  DataStoreName=EHBMotor_Pos_AD  DataStoreElements=EHBMotor_Pos_AD  IndexOptions=Index vector (dialog)  Indices=1  OutputSizes=1
  Data Store Read7 : DataStoreRead  DataStoreName=EHBMotor_PWM  DataStoreElements=EHBMotor_PWM  IndexOptions=Index vector (dialog)  Indices=1  OutputSizes=1
  Motor_Angle : Outport  VectorParamsAs1DForOutWhenUnconnected=off
  Motor_actPWM : Outport  Port=2  VectorParamsAs1DForOutWhenUnconnected=off
  wires:
  Data Store Read7/1 -> Motor_actPWM/1
  Data Store Read4/1 -> Motor_Angle/1

== system EHB_MOTOR/EHB_MOTOR_PRO/INPUT/OUTPUT2INPUT ==
  LAST_OUTPUT : Inport
  Feedback : Outport  VectorParamsAs1DForOutWhenUnconnected=off
  wires:
  LAST_OUTPUT/1 -> Feedback/1

== system EHB_MOTOR/EHB_MOTOR_PRO/MODE/KL15_condition ==
  INPUT_BUS : Inport
  Bus Selector : BusSelector  OutputSignals=AI_BUS.EHB_vKL15_filtered
  Constant : Constant  Value=9
  Relational Operator : RelationalOperator  OutDataTypeStr=boolean  RndMeth=Simplest  InputSameDT=off
  ignition_status : Outport  VectorParamsAs1DForOutWhenUnconnected=off
  wires:
  INPUT_BUS/1 -> Bus Selector/1
  Bus Selector/1 -> Relational Operator/1  "<EHB_vKL15_filtered>"
  Constant/1 -> Relational Operator/2
  Relational Operator/1 -> ignition_status/1

== system EHB_MOTOR/EHB_MOTOR_PRO/MODE/Subsystem ==
  INPUT_BUS : Inport
  Bus Selector : BusSelector  OutputSignals=Feedback.DIAG_DELAY.EHBVoltageLow2,Feedback.DIAG_DELAY.EHBVoltageHigh2,Feedback.DIAG_DELAY.TempSensorOverride,Feedback.DIAG_DELAY.Chip7189_err,Feedback.DIAG_DELAY.PressureSensorERR
  Compare To Zero{,1..4} (5 alike) : simulink/Logic and Bit Operations/Compare To Zero  relop===  OutDataTypeStr=boolean
  Logical Operator : Logic  Inputs=5  AllPortsSameDT=off  OutDataTypeStr=boolean
  Logical Operator1 : Logic  Operator=NOT  AllPortsSameDT=off  OutDataTypeStr=boolean
  Fault_Status : Outport  VectorParamsAs1DForOutWhenUnconnected=off
  wires:
  INPUT_BUS/1 -> Bus Selector/1
  Bus Selector/1 -> Compare To Zero/1  "<EHBVoltageLow2>"
  Bus Selector/2 -> Compare To Zero1/1  "<EHBVoltageHigh2>"
  Bus Selector/3 -> Compare To Zero2/1  "<TempSensorOverride>"
  Bus Selector/4 -> Compare To Zero3/1  "<Chip7189_err>"
  Bus Selector/5 -> Compare To Zero4/1  "<PressureSensorERR>"
  Compare To Zero/1 -> Logical Operator/1
  Compare To Zero1/1 -> Logical Operator/2
  Compare To Zero2/1 -> Logical Operator/3
  Compare To Zero3/1 -> Logical Operator/4
  Compare To Zero4/1 -> Logical Operator/5
  Logical Operator/1 -> Logical Operator1/1
  Logical Operator1/1 -> Fault_Status/1

== system EHB_MOTOR/EHB_MOTOR_PRO/Motor_ESTIMATE/Motor_Length ==
  In1 : Inport
  EHB_Mot_length : Outport  VectorParamsAs1DForOutWhenUnconnected=off
  wires:
  In1/1 -> EHB_Mot_length/1

== system EHB_MOTOR/EHB_MOTOR_PRO/Motor_ESTIMATE/Motor_Temp ==
  In1 : Inport
  EHB_Mot_temp : Outport  VectorParamsAs1DForOutWhenUnconnected=off
  wires:
  In1/1 -> EHB_Mot_temp/1

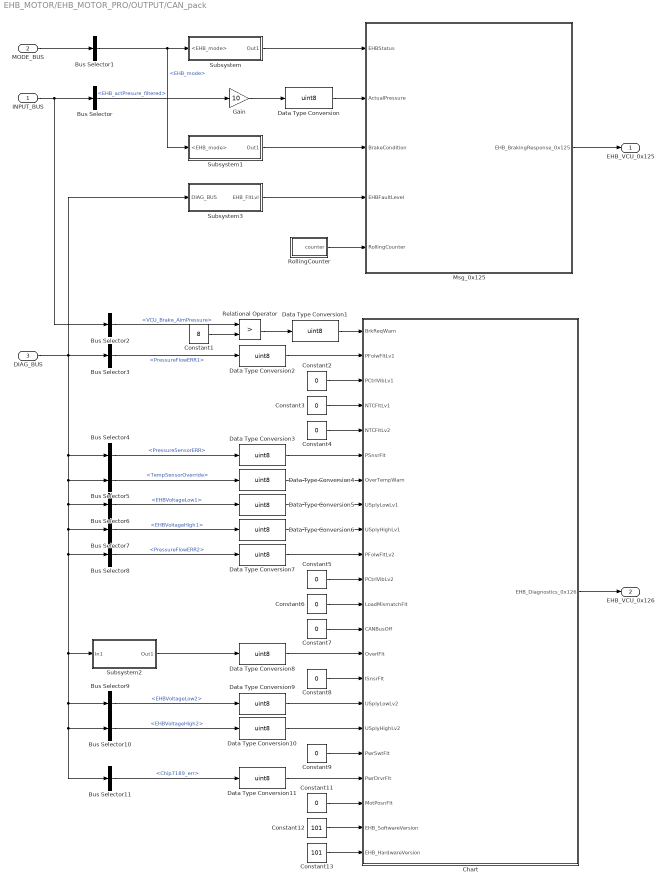
== system EHB_MOTOR/EHB_MOTOR_PRO/OUTPUT/CAN_pack ==
  INPUT_BUS : Inport
  MODE_BUS : Inport  Port=2
  DIAG_BUS : Inport  Port=3
  Bus Selector : BusSelector  OutputSignals=AI_BUS.EHB_actPresure_filtered
  Bus Selector1 : BusSelector  OutputSignals=EHB_mode
  Bus Selector10 : BusSelector  OutputSignals=EHBVoltageHigh2
  Bus Selector11 : BusSelector  OutputSignals=Chip7189_err
  Bus Selector2 : BusSelector  OutputSignals=CAN_BUS.VCU_Brake_AimPressure
  Bus Selector3 : BusSelector  OutputSignals=PressureFlowERR1
  Bus Selector4 : BusSelector  OutputSignals=PressureSensorERR
  Bus Selector5 : BusSelector  OutputSignals=TempSensorOverride
  Bus Selector6 : BusSelector  OutputSignals=EHBVoltageLow1
  Bus Selector7 : BusSelector  OutputSignals=EHBVoltageHigh1
  Bus Selector8 : BusSelector  OutputSignals=PressureFlowERR2
  Bus Selector9 : BusSelector  OutputSignals=EHBVoltageLow2
  Chart : Stateflow chart  TreatAsAtomicUnit=on
  Constant1 : Constant  Value=8  OutDataTypeStr=Inherit: Inherit via back propagation
  Constant{2..9,11} (9 alike) : Constant  Value=0  OutDataTypeStr=uint8
  Constant12 : Constant  Value=101  OutDataTypeStr=uint8
  Constant13 : Constant  Value=101  OutDataTypeStr=uint8
  Data Type Conversion{,1..11} (12 alike) : DataTypeConversion  OutDataTypeStr=uint8  SaturateOnIntegerOverflow=off  RndMeth=Floor
  Gain : Gain  Gain=10
  Msg_0x125 : Stateflow chart  TreatAsAtomicUnit=on
  Relational Operator : RelationalOperator  Operator=>  OutDataTypeStr=boolean  RndMeth=Simplest  InputSameDT=off
  RollingCounter : Stateflow chart  TreatAsAtomicUnit=on
  Subsystem : Subsystem
  Subsystem1 : Subsystem
  Subsystem2 : Subsystem
  Subsystem3 : Subsystem
  EHB_VCU_0x125 : Outport  VectorParamsAs1DForOutWhenUnconnected=off
  EHB_VCU_0x126 : Outport  Port=2  VectorParamsAs1DForOutWhenUnconnected=off
  wires:
  Msg_0x125/1(EHB_BrakingResponse_0x125) -> EHB_VCU_0x125/1
  INPUT_BUS/1 -> Bus Selector/1, Bus Selector2/1
  MODE_BUS/1 -> Bus Selector1/1
  Bus Selector/1 -> Gain/1  "<EHB_actPresure_filtered>"
  Gain/1 -> Data Type Conversion/1
  Bus Selector1/1 -> Subsystem/1(<EHB_mode>), Subsystem1/1(<EHB_mode>)  "<EHB_mode>"
  Subsystem/1(Out1) -> Msg_0x125/1(EHBStatus)
  Subsystem1/1(Out1) -> Msg_0x125/3(BrakeCondition)
  Data Type Conversion/1 -> Msg_0x125/2(ActualPressure)
  RollingCounter/1(counter) -> Msg_0x125/5(RollingCounter)
  Subsystem3/1(EHB_FltLvl) -> Msg_0x125/4(EHBFaultLevel)
  Bus Selector2/1 -> Relational Operator/1  "<VCU_Brake_AimPressure>"
  Constant1/1 -> Relational Operator/2
  Relational Operator/1 -> Data Type Conversion1/1
  Data Type Conversion1/1 -> Chart/1(BrkReqWarn)
  Chart/1(EHB_Diagnostics_0x126) -> EHB_VCU_0x126/1
  DIAG_BUS/1 -> Subsystem3/1(DIAG_BUS), Bus Selector4/1, Bus Selector5/1, Bus Selector6/1, Bus Selector7/1, Bus Selector8/1, Subsystem2/1(In1), Bus Selector10/1, Bus Selector11/1, Bus Selector9/1, Bus Selector3/1
  Bus Selector3/1 -> Data Type Conversion2/1  "<PressureFlowERR1>"
  Constant2/1 -> Chart/3(PCtrlVibLv1)
  Constant3/1 -> Chart/4(NTCFltLv1)
  Constant4/1 -> Chart/5(NTCFltLv2)
  Bus Selector4/1 -> Data Type Conversion3/1  "<PressureSensorERR>"
  Data Type Conversion2/1 -> Chart/2(PFolwFltLv1)
  Data Type Conversion3/1 -> Chart/6(PSnsrFlt)
  Bus Selector5/1 -> Data Type Conversion4/1  "<TempSensorOverride>"
  Data Type Conversion4/1 -> Chart/7(OverTempWarn)
  Bus Selector6/1 -> Data Type Conversion5/1  "<EHBVoltageLow1>"
  Bus Selector7/1 -> Data Type Conversion6/1  "<EHBVoltageHigh1>"
  Bus Selector8/1 -> Data Type Conversion7/1  "<PressureFlowERR2>"
  Constant5/1 -> Chart/11(PCtrlVibLv2)
  Constant6/1 -> Chart/12(LoadMismatchFlt)
  Constant7/1 -> Chart/13(CANBusOff)
  Constant8/1 -> Chart/15(ISnsrFlt)
  Bus Selector9/1 -> Data Type Conversion9/1  "<EHBVoltageLow2>"
  Bus Selector10/1 -> Data Type Conversion10/1  "<EHBVoltageHigh2>"
  Data Type Conversion5/1 -> Chart/8(USplyLowLv1)
  Data Type Conversion6/1 -> Chart/9(USplyHighLv1)
  Data Type Conversion7/1 -> Chart/10(PFolwFltLv2)
  Subsystem2/1(Out1) -> Data Type Conversion8/1
  Data Type Conversion9/1 -> Chart/16(USplyLowLv2)
  Data Type Conversion10/1 -> Chart/17(USplyHighLv2)
  Constant9/1 -> Chart/18(PwrSwtFlt)
  Bus Selector11/1 -> Data Type Conversion11/1  "<Chip7189_err>"
  Constant11/1 -> Chart/20(MotPosnFlt)
  Data Type Conversion8/1 -> Chart/14(OverIFlt)
  Constant12/1 -> Chart/21(EHB_SoftwareVersion)
  Constant13/1 -> Chart/22(EHB_HardwareVersion)
  Data Type Conversion11/1 -> Chart/19(PwrDrvrFlt)
